simulink model "DT_Linear_n9960210"  (R2021a)
settings: Solver=VariableStepAuto  StartTime=0.0  StopTime=10.0  RelTol=1e-3
values from neighbouring files (symbols this model uses):
  u_bar = 1    [main_n9960210_plotall.m]
  x_bar = [2*u_bar-1 ... (first row only)    [main_n9960210_plotall.m]
undefined symbols (not defined in the file or in its folder): Ad, Bd, Cd, Dd, Kd, Ts, x0_tilde
settings Model: Creator=isaac  LastModifiedBy=isaac

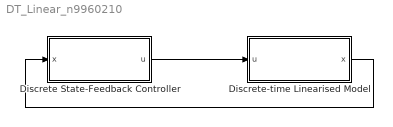
== system DT_Linear_n9960210 ==
  Discrete State-Feedback Controller : Subsystem
  Discrete-time Linearised Model : Subsystem
  wires:
  Discrete-time Linearised Model/1(x) -> Discrete State-Feedback Controller/1(x)
  Discrete State-Feedback Controller/1(u) -> Discrete-time Linearised Model/1(u)

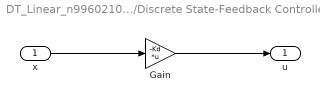
== system DT_Linear_n9960210/Discrete State-Feedback Controller ==
  x : Inport
  Gain : Gain  Gain=-Kd  Multiplication=Matrix(K*u)
  u : Outport
  wires:
  x/1 -> Gain/1
  Gain/1 -> u/1

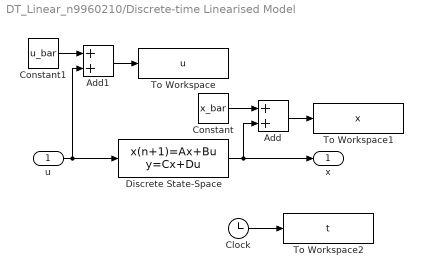
== system DT_Linear_n9960210/Discrete-time Linearised Model ==
  u : Inport
  Add : Sum
  Add1 : Sum
  Clock : Clock
  Constant : Constant  Value=x_bar
  Constant1 : Constant  Value=u_bar
  Discrete State-Space : DiscreteStateSpace  A=Ad  B=Bd  C=Cd  D=Dd  InitialCondition=x0_tilde  SampleTime=Ts
  To Workspace : ToWorkspace  VariableName=u  SampleTime=Ts
  To Workspace1 : ToWorkspace  VariableName=x  SampleTime=Ts
  To Workspace2 : ToWorkspace  VariableName=t  SampleTime=Ts
  x : Outport
  wires:
  u/1 -> Add1/2, Discrete State-Space/1
  Clock/1 -> To Workspace2/1
  Discrete State-Space/1 -> Add/2, x/1
  Constant/1 -> Add/1
  Add/1 -> To Workspace1/1
  Constant1/1 -> Add1/1
  Add1/1 -> To Workspace/1
